simulink library "mechanics"  (R2013a)
settings: Solver=ode45  StartTime=0.0  StopTime=10.0  FixedStep=0.02  RelTol=1e-3
undefined symbols (not defined in the file): magnitude
settings Model: Creator=Goh  LastModifiedBy=Goh

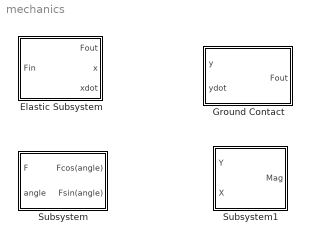
== system mechanics ==
  Elastic Subsystem : Subsystem  mask(Elastic Model){m=0, k=0, c=0}
      mask prompts: m "Mass [kg]"; k "Stiffness [N/m]"; c "Damping [Ns/m]"
      mask help: Elastic model allows user to input the amount of force applied to an elastic system. The output will be the time response of the system.
  Ground Contact : Subsystem  mask(Ground contact){k=0, c=0}
      mask prompts: k "Stiffness Coefficient  [N/m]"; c "Damping Coefficient [Ns/m]"
      mask help: Ground contact subsystem represent a basic spring-mass model as contact ground. Output is the normal force based on depth and depth penetration
  Subsystem : Subsystem
  Subsystem1 : Subsystem  mask(Magnitude of Two Lengths){}
      mask help: This block outputs the diagonal length of two lengths perpendicular to each other

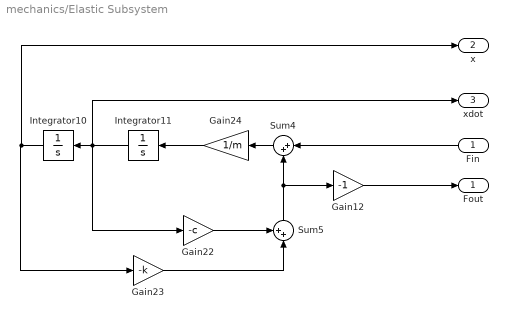
== system mechanics/Elastic Subsystem ==
  Fin : Inport
  Gain12 : Gain  Gain=-1
  Gain22 : Gain  Gain=-c
  Gain23 : Gain  Gain=-k
  Gain24 : Gain  Gain=1/m
  Integrator10 : Integrator
  Integrator11 : Integrator
  Sum4 : Sum  Inputs=|++
  Sum5 : Sum  Inputs=++|
  Fout : Outport
  x : Outport  Port=2
  xdot : Outport  Port=3
  wires:
  Integrator11/1 -> xdot/1, Gain22/1, Integrator10/1
  Fin/1 -> Sum4/1
  Gain24/1 -> Integrator11/1
  Gain22/1 -> Sum5/1
  Sum5/1 -> Sum4/2, Gain12/1
  Gain23/1 -> Sum5/2
  Gain12/1 -> Fout/1
  Sum4/1 -> Gain24/1
  Integrator10/1 -> x/1, Gain23/1

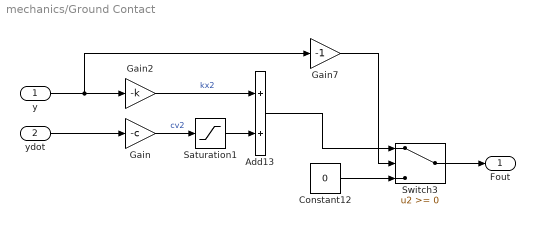
== system mechanics/Ground Contact ==
  y : Inport
  ydot : Inport  Port=2
  Add13 : Sum
  Constant12 : Constant  Value=0
  Gain : Gain  Gain=-c
  Gain2 : Gain  Gain=-k
  Gain7 : Gain  Gain=-1
  Saturation1 : Saturate  UpperLimit=inf  LowerLimit=0
  Switch3 : Switch
  Fout : Outport
  wires:
  Switch3/1 -> Fout/1
  Gain2/1 -> Add13/1  "kx2"
  y/1 -> Gain7/1, Gain2/1
  Constant12/1 -> Switch3/3
  Saturation1/1 -> Add13/2
  Gain/1 -> Saturation1/1  "cv2"
  Gain7/1 -> Switch3/2
  Add13/1 -> Switch3/1
  ydot/1 -> Gain/1

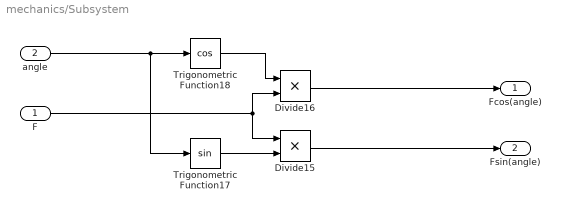
== system mechanics/Subsystem ==
  F : Inport
  angle : Inport  Port=2
  Divide15 : Product  Inputs=**
  Divide16 : Product  Inputs=**
  Trigonometric Function17 : Trigonometry
  Trigonometric Function18 : Trigonometry  Operator=cos
  Fcos(angle) : Outport
  Fsin(angle) : Outport  Port=2
  wires:
  Trigonometric Function18/1 -> Divide16/1
  angle/1 -> Trigonometric Function17/1, Trigonometric Function18/1
  Divide16/1 -> Fcos(angle)/1
  F/1 -> Divide16/2, Divide15/1
  Trigonometric Function17/1 -> Divide15/2
  Divide15/1 -> Fsin(angle)/1

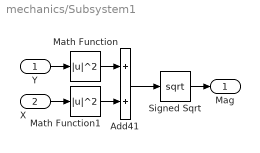
== system mechanics/Subsystem1 ==
  Y : Inport
  X : Inport  Port=2
  Add41 : Sum
  Math Function : Math  Operator=magnitude^2  SaturateOnIntegerOverflow=on
  Math Function1 : Math  Operator=magnitude^2  SaturateOnIntegerOverflow=on
  Signed Sqrt : Sqrt  SaturateOnIntegerOverflow=on
  Mag : Outport
  wires:
  Y/1 -> Math Function/1
  Signed Sqrt/1 -> Mag/1
  X/1 -> Math Function1/1
  Math Function1/1 -> Add41/2
  Math Function/1 -> Add41/1
  Add41/1 -> Signed Sqrt/1
